simulink model "with_controller"  (R2020a)
settings: Solver=VariableStepAuto  StartTime=0.0  StopTime=5  RelTol=1e-3
values from neighbouring files (symbols this model uses):
  alpha0 = 1.26623672724    [controller_aero_data.mat]
  c = 4    [aerodata.mat]    (also in controller_aero_data.mat)
  CD = [0.02311 0.024258 0.025763 0.027458 0.029228 0.032142 0.036767 0.043354 0.054016 0.019425 0.021643 0.02423 ... (27 elements, 9x3)]    [aerodata.mat]    (also in controller_aero_data.mat)
  CL = [0.060978 0.158725 0.256402 0.353948 0.451302 0.548404 0.645194 0.741612 0.8376 0.140071 0.23768 0.335161 ... (27 elements, 9x3)]    [aerodata.mat]    (also in controller_aero_data.mat)
  CM = [0.496711 0.453087 0.40838 0.362641 0.315812 0.268147 0.219899 0.171225 0.122257 0.032141 -0.010092 -0.053151 ... (27 elements, 9x3)]    [aerodata.mat]    (also in controller_aero_data.mat)
  Cmq = -0.988397408697    [controller_aero_data.mat]
  g = 32.174    [aerodata.mat]    (also in controller_aero_data.mat)
  gamma0 = -4.93316661608    [controller_aero_data.mat]
  S = 1.33333333333    [aerodata.mat]    (also in controller_aero_data.mat)
libraries: simulink_extras x3, simulink x2, aerolib3dof2 x1, aerolibatmos2 x1, aerolibasang x1, aerolibactuator x1, sldrtlib x1
settings Model: Creator=Khojasteh Mirza  LastModifiedBy=Khojasteh Mirza
settings SolverCC: ZeroCrossAlgorithm=Adaptive
settings DebuggingCC: IgnoredZcDiagnostic=none

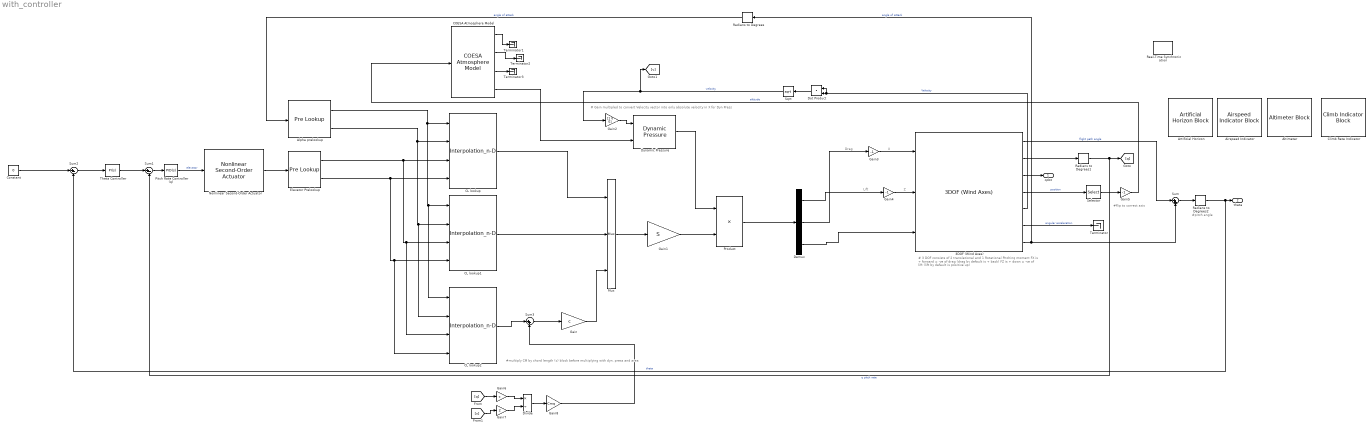
== system with_controller ==
  note: # Gain multipled to convert Velocity vector into only absolute velocity in X for Dyn Press
  note: X
  note: #flip to correct axis
  note: #pitch angle
  note: Drag
  note: # 3 DOF consists of 2 translational and 1 Rotational Pitching moment
      | FX is + forward = -ve of drag (drag by default is + back)
      | FZ is + down = -ve of lift (lift by default is positive up)
  note: Z
  note: #multiply CM by chord length (c) block before multiplying with dyn. press and area
  note: Lift
  3DOF (Wind Axes) : aerolib3dof2/3DOF (Wind Axes)  units=English (Velocity in ft/s)  mtype=Fixed  V_ini=v0  alpha_ini=deg2rad(alpha0)  gamma_ini=deg2rad(gamma0)  q_ini=0  pos_ini=[0 -10000]  mass=m  mass_e=0.5  mass_f=3.0  Iyy=Iyy  Iyy_e=0.5  Iyy_f=3.0  g_in=Internal  g=g  vre_flag=on  abi_flag=off  V_statename=''  alpha_statename=''  gamma_statename=''  q_statename=''  pos_statename=''  mass_statename=''
      settings: SourceProductBaseCode=AE
  Airspeed Indicator : AirspeedIndicatorBlock  ScaleMin=0  ScaleMax=120
  Alpha prelookup : PreLookup  BreakpointsData=alpha  ExtrapMethod=Linear
  Altimeter : AltimeterBlock
  Artificial Horizon : ArtificialHorizonBlock
  CL lookup : Interpolation_n-D  Table=CL  InternalRulePriority=Speed
  CL lookup1 : Interpolation_n-D  Table=CD  InternalRulePriority=Speed
  CL lookup2 : Interpolation_n-D  Table=CM  InternalRulePriority=Speed
  COESA Atmosphere Model : aerolibatmos2/COESA Atmosphere Model  units=English (Velocity in ft/s)  spec=1976 COESA-extended U.S. Standard Atmosphere  model=Profile  profile_var=High temperature  profile_percent=1%  profile_alt=5 km (16404 ft)  envelope_var=High temperature  envelope_percent=1%  action=Warning
  Climb Rate Indicator : ClimbIndicatorBlock  ScaleMax=40
  Constant : Constant  Value=0
  Demux : Demux  Outputs=3
  Divide : Product  Inputs=*/
  Dot Product : DotProduct  InputSameDT=on  OutDataTypeStr=Inherit: Inherit via internal rule
  Dynamic Pressure : aerolibasang/Dynamic Pressure
  Elevator Prelookup : PreLookup  BreakpointsData=elevator  ExtrapMethod=Linear
  Gain : Gain  Gain=c
  Gain1 : Gain  Gain=S
  Gain2 : Gain  Gain=[1 0 0]
  Gain3 : Gain  Gain=-1
  Gain4 : Gain  Gain=-1
  Gain5 : Gain  Gain=-1
  Gain6 : Gain  Gain=c
  Gain7 : Gain  Gain=2
  Gain8 : Gain  Gain=Cmq
  Mux : Mux  Inputs=3
  Nonlinear Second-Order Actuator : aerolibactuator/Nonlinear Second-Order Actuator  wn_fin=60  z_fin=0.7  fin_max=25  fin_min=-25  fin_maxrate=180  fin_act_0=0  fin_act_vel=0
      settings: SourceProductBaseCode=AE
  Pitch Rate Controller (q) : simulink/Continuous/PID Controller  Controller=PID  Form=Parallel  TimeDomain=Continuous-time  UseExternalTs=off  SampleTime=-1  IntegratorMethod=Forward Euler  FilterMethod=Forward Euler  ControllerParametersSource=internal  P=-0.159438011245571  I=-0.189887826544235  D=0.0401106364592781  UseFilter=on  N=3.97495590496148  TunerSelectOption=Transfer Function Based (PID Tuner App)  InitialConditionSource=internal  InitialConditionForIntegrator=0  InitialConditionForFilter=0  DifferentiatorICPrevScaledInput=0  ExternalReset=none  TrackingMode=off  Kt=1  LimitOutput=off  UpperSaturationLimit=inf  LowerSaturationLimit=-inf  LinearizeAsGain=on  AntiWindupMode=none  Kb=1  POutMin=[]  POutMax=[]  IOutMin=[]  IOutMax=[]  DOutMin=[]  DOutMax=[]  NOutMin=[]  NOutMax=[]  SumOutMin=[]  SumOutMax=[]  SaturationOutMin=[]  SaturationOutMax=[]  PParamMin=[]  PParamMax=[]  IParamMin=[]  IParamMax=[]  DParamMin=[]  DParamMax=[]  NParamMin=[]  NParamMax=[]  KbParamMin=[]  KbParamMax=[]  KtParamMin=[]  KtParamMax=[]  KbOutMin=[]  KbOutMax=[]  KtOutMin=[]  KtOutMax=[]  IntegratorOutMin=[]  IntegratorOutMax=[]  FilterOutMin=[]  FilterOutMax=[]  SumI1OutMin=[]  SumI1OutMax=[]  SumI2OutMin=[]  SumI2OutMax=[]  SumI3OutMin=[]  SumI3OutMax=[]  SumI4OutMin=[]  SumI4OutMax=[]  SumDOutMin=[]  SumDOutMax=[]  DifferentiatorOutMin=[]  DifferentiatorOutMax=[]  FilterDiffOutCoefMin=[]  FilterDiffOutCoefMax=[]  ReciprocalOutMin=[]  ReciprocalOutMax=[]  SumDenOutMin=[]  SumDenOutMax=[]  SumNumOutMin=[]  SumNumOutMax=[]  DivideOutMin=[]  DivideOutMax=[]  UdiffTsProdOutMin=[]  UdiffTsProdOutMax=[]  NTsProdOutMin=[]  NTsProdOutMax=[]  UintegralTsProdOutMin=[]  UintegralTsProdOutMax=[]  UngainTsProdOutMin=[]  UngainTsProdOutMax=[]  IntegratorContinuousStateAttributes=''  IntegratorStateMustResolveToSignalObject=off  IntegratorRTWStateStorageClass=Auto  FilterContinuousStateAttributes=''  FilterStateMustResolveToSignalObject=off  FilterRTWStateStorageClass=Auto  ParallelPVariant=InternalParameters  IdealPVariant=Disabled  IVariant=InternalParameters  DVariant=InternalParameters  IntegratorVariant=Continuous  SatVariant=Disabled  AWVariant=Passthrough  PCopyVariant=Disabled  TRVariant=Disabled  FdbkBlocksVariant=Forward  IdealPFdbkVariant=Disabled  SatFdbkVariant=Disabled  DerivativeFilterVariant=ContFilter  NVariant=InternalParameters  NCopyVariant=Disabled  FilterICVariant=InternalICsFilter  IntegratorICVariant=InternalICs  ExternalResetVariant=Disabled  TRSumVariant=Passthrough  SumFdbkVariant=Disabled  SumVariant=Sum_PID  TsampFilterVariant=InternalTs  TsampNgainVariant=Passthrough  TsampIntegralVariant=Passthrough
  Product : Product
  Radians to Degrees : simulink_extras/Transformations/Radians to Degrees
  Radians to Degrees1 : simulink_extras/Transformations/Radians to Degrees
  Radians to Degrees2 : simulink_extras/Transformations/Radians to Degrees
  Real-Time Synchronization : sldrtlib/Real-Time Synchronization  SampleTime=1.0  MaxMissedTicks=100000  ShowMissedTicks=on  YieldWhenWaiting=off
  Selector : Selector  InputPortWidth=2  IndexOptions=Index vector (dialog)  Indices=2  OutputSizes=1
  Sqrt : Sqrt  SaturateOnIntegerOverflow=on
  Sum : Sum  Inputs=|++
  Sum1 : Sum  Inputs=|+-
  Sum2 : Sum  Inputs=|+-
  Sum3 : Sum  Inputs=|++
  Terminator{,1..3} (4 alike) : Terminator
  Theta Controller : simulink/Continuous/PID Controller  Controller=PI  Form=Parallel  TimeDomain=Continuous-time  UseExternalTs=off  SampleTime=-1  IntegratorMethod=Forward Euler  FilterMethod=Forward Euler  ControllerParametersSource=internal  P=1.02628820194674  I=0.620181090339484  D=-0.000170815291052217  UseFilter=on  N=11986.5442584726  TunerSelectOption=Transfer Function Based (PID Tuner App)  InitialConditionSource=internal  InitialConditionForIntegrator=0  InitialConditionForFilter=0  DifferentiatorICPrevScaledInput=0  ExternalReset=none  TrackingMode=off  Kt=1  LimitOutput=off  UpperSaturationLimit=inf  LowerSaturationLimit=-inf  LinearizeAsGain=on  AntiWindupMode=none  Kb=1  POutMin=[]  POutMax=[]  IOutMin=[]  IOutMax=[]  DOutMin=[]  DOutMax=[]  NOutMin=[]  NOutMax=[]  SumOutMin=[]  SumOutMax=[]  SaturationOutMin=[]  SaturationOutMax=[]  PParamMin=[]  PParamMax=[]  IParamMin=[]  IParamMax=[]  DParamMin=[]  DParamMax=[]  NParamMin=[]  NParamMax=[]  KbParamMin=[]  KbParamMax=[]  KtParamMin=[]  KtParamMax=[]  KbOutMin=[]  KbOutMax=[]  KtOutMin=[]  KtOutMax=[]  IntegratorOutMin=[]  IntegratorOutMax=[]  FilterOutMin=[]  FilterOutMax=[]  SumI1OutMin=[]  SumI1OutMax=[]  SumI2OutMin=[]  SumI2OutMax=[]  SumI3OutMin=[]  SumI3OutMax=[]  SumI4OutMin=[]  SumI4OutMax=[]  SumDOutMin=[]  SumDOutMax=[]  DifferentiatorOutMin=[]  DifferentiatorOutMax=[]  FilterDiffOutCoefMin=[]  FilterDiffOutCoefMax=[]  ReciprocalOutMin=[]  ReciprocalOutMax=[]  SumDenOutMin=[]  SumDenOutMax=[]  SumNumOutMin=[]  SumNumOutMax=[]  DivideOutMin=[]  DivideOutMax=[]  UdiffTsProdOutMin=[]  UdiffTsProdOutMax=[]  NTsProdOutMin=[]  NTsProdOutMax=[]  UintegralTsProdOutMin=[]  UintegralTsProdOutMax=[]  UngainTsProdOutMin=[]  UngainTsProdOutMax=[]  IntegratorContinuousStateAttributes=''  IntegratorStateMustResolveToSignalObject=off  IntegratorRTWStateStorageClass=Auto  FilterContinuousStateAttributes=''  FilterStateMustResolveToSignalObject=off  FilterRTWStateStorageClass=Auto  ParallelPVariant=InternalParameters  IdealPVariant=Disabled  IVariant=InternalParameters  DVariant=Disabled  IntegratorVariant=Continuous  SatVariant=Disabled  AWVariant=Passthrough  PCopyVariant=Disabled  TRVariant=Disabled  FdbkBlocksVariant=Forward  IdealPFdbkVariant=Disabled  SatFdbkVariant=Disabled  DerivativeFilterVariant=Disabled  NVariant=Disabled  NCopyVariant=Disabled_SignalSpec  FilterICVariant=Disabled  IntegratorICVariant=InternalICs  ExternalResetVariant=Disabled  TRSumVariant=Passthrough  SumFdbkVariant=Disabled  SumVariant=Sum_PI  TsampFilterVariant=InternalTs  TsampNgainVariant=Passthrough  TsampIntegralVariant=Passthrough
  qdot : Outport
  theta : Outport  Port=2
  wires:
  3DOF (Wind Axes)/6 -> Terminator/1  "angular acceleration"
  3DOF (Wind Axes)/2 -> Radians to Degrees1/1
  3DOF (Wind Axes)/1 -> Sum/1  "flight path angle"
  Demux/2 -> Gain3/1
  3DOF (Wind Axes)/7 -> Sum/2, Radians to Degrees/1  "angle of attack"
  Gain1/1 -> Product/2
  Sum/1 -> Radians to Degrees2/1
  Selector/1 -> Gain5/1
  Gain/1 -> Mux/3
  Gain2/1 -> Dynamic Pressure/1
  Mux/1 -> Gain1/1
  Radians to Degrees/1 -> Alpha prelookup/1  "angle of attack"
  Gain4/1 -> 3DOF (Wind Axes)/2
  Gain5/1 -> COESA Atmosphere Model/1  "altitude"
  Demux/1 -> Gain4/1
  CL lookup/1 -> Mux/1
  3DOF (Wind Axes)/4 -> Selector/1  "position"
  COESA Atmosphere Model/4 -> Dynamic Pressure/2
  Demux/3 -> 3DOF (Wind Axes)/3
  3DOF (Wind Axes)/3 -> qdot/1
  Alpha prelookup/2 -> CL lookup2/2, CL lookup1/2, CL lookup/2
  Elevator Prelookup/1 -> CL lookup2/3, CL lookup1/3, CL lookup/3
  CL lookup1/1 -> Mux/2
  Elevator Prelookup/2 -> CL lookup2/4, CL lookup1/4, CL lookup/4
  Dynamic Pressure/1 -> Product/1
  Alpha prelookup/1 -> CL lookup2/1, CL lookup1/1, CL lookup/1
  3DOF (Wind Axes)/5 -> Dot Product/1, Dot Product/2  "Velocity"
  Product/1 -> Demux/1
  Dot Product/1 -> Sqrt/1
  Radians to Degrees1/1 -> [q], Sum1/2  "q pitch rate"
  Gain3/1 -> 3DOF (Wind Axes)/1
  Sqrt/1 -> [v], Gain2/1  "velocity"
  Sum1/1 -> Pitch Rate Controller (q)/1
  Pitch Rate Controller (q)/1 -> Nonlinear Second-Order Actuator/1  "elevator"
  Constant/1 -> Sum2/1
  Sum2/1 -> Theta Controller/1
  Radians to Degrees2/1 -> Sum2/2, theta/1  "theta"
  Nonlinear Second-Order Actuator/1 -> Elevator Prelookup/1
  Theta Controller/1 -> Sum1/1
  CL lookup2/1 -> Sum3/1
  Sum3/1 -> Gain/1
  COESA Atmosphere Model/1 -> Terminator1/1
  COESA Atmosphere Model/2 -> Terminator2/1
  COESA Atmosphere Model/3 -> Terminator3/1
  [q] -> Gain6/1
  [v] -> Gain7/1
  Gain7/1 -> Divide/2
  Gain6/1 -> Divide/1
  Divide/1 -> Gain8/1
  Gain8/1 -> Sum3/2
